simulink model "Quaternions_Method_main"  (R2021b)
settings: Solver=ode4  StartTime=0.0  StopTime=Time  FixedStep=1e-2  RelTol=1e-13  AbsTol=1e-8
values from neighbouring files (symbols this model uses):
  a = 8.6251e+06    (= 8625100)    [Main.m]
  c = 299792*10^3    (= 299792000)    [Main.m]
  e = 0.1195    [Main.m]
  f_mag = 18    [Main.m]
  H_0 = sqrt((g_1_0)^2 + (g_1_1)^2 + (h_1_1)^2)    [Main.m]
  i = 0.3815    [Main.m]
  MB = [2000; 0.3; 1; 0.12].*1e-2    [Main.m]
  muP = G*Mt    (= 398527110340000)    [Main.m]
  omega_0 = [om_x, om_y, om_z]    [Main.m]
  p_acc = 0.5    [Main.m]
  RD = 0.1*ones(1,10)    [Main.m]
  RS_MB = 0.5    [Main.m]
  RS_SP = 0.1    [Main.m]
  SP = [2000; 0.3; 1; 0.12].*1e-2    [Main.m]
  theta0 = 0    [Main.m]
  w_E = (2*pi)/(24*3600)    (= 7.27220521664e-05)    [Main.m]
undefined symbols (not defined in the file or in its folder): A_BN_0, A_rw, A_rw_star, k1, k2, magnitude, mr, sig_b, sig_n, T, t_sample
libraries: matrix_library x15, vrlib x8, simulink x2, simulink_extras x1
(part 5 of 5)

== system Quaternions_Method_main/Enviroment/Solar Radiation Perturbation/Sum forces/determine highlighted area/creazione della matrice che ha per colonne i vettori distanza tra il CM del MB e i centri geom delle aree illuminate dal sole /creazione raggi vettore tra CM MB e centro facce illuminate della faccia che ha come normale l'asse k/If Action Subsystem4 ==
  Areas_vect : Inport
  MB1 : Inport  Port=2
  Action Port : ActionPort  ActionPortLabel=if(u1<0 & u2>0)
  Add : Sum  Inputs=+|-
  Add1 : Sum  Inputs=+|-
  Add2 : Sum
  Demux : Demux  Outputs=3
  Demux1 : Demux  Outputs=3
  Demux2 : Demux
  Divide : Product  Inputs=*/
  Divide1 : Product  Inputs=*/
  Gain{,1..3} (4 alike) : Gain  Gain=1/2
  Gain4 : Gain  Gain=-1
  Ground : Ground
  Ground1 : Ground
  Mux : Mux  Inputs=3
  Mux1 : Mux  Inputs=3
  Reshape{,1..3} (4 alike) : Reshape  OutputDimensionality=Column vector (2-D)
  Terminator{,1..3,8..9} (6 alike) : Terminator
  r_cface_cluce_xneg_y_pos : Outport
  wires:
  Demux/2 -> Terminator8/1
  Demux/1 -> Terminator9/1
  Demux1/2 -> Terminator1/1
  Demux1/1 -> Terminator/1
  Add2/1 -> r_cface_cluce_xneg_y_pos/1
  Reshape3/1 -> Add2/2
  Reshape2/1 -> Add2/1
  Divide1/1 -> Gain3/1
  Reshape1/1 -> Demux1/1
  Gain2/1 -> Add1/1
  Gain3/1 -> Add1/2
  Demux1/3 -> Divide1/1
  Ground/1 -> Mux1/1, Mux1/3
  Mux1/1 -> Reshape3/1  "raggio vettore che collega il centro geom della faccia con il centro geom della faccia illuminata dal sole lungo j"
  Reshape/1 -> Demux/1
  Ground1/1 -> Mux/2, Mux/3
  Areas_vect/1 -> Reshape1/1, Reshape/1
  Gain/1 -> Add/1
  Demux/3 -> Divide/1
  Gain1/1 -> Add/2
  Mux/1 -> Reshape2/1  "raggio vettore che collega il centro geom della faccia con il centro geom della faccia illuminata dal sole lungo -i"
  Divide/1 -> Gain1/1
  [b_MB] -> Divide/2
  [a_MB] -> Gain/1
  Add/1 -> Gain4/1
  Gain4/1 -> Mux/1
  Add1/1 -> Mux1/2
  [b_MB] -> Gain2/1
  [a_MB] -> Divide1/2
  Demux2/1 -> Terminator2/1
  Demux2/2 -> [a_MB]
  MB1/1 -> Demux2/1
  Demux2/3 -> [b_MB]
  Demux2/4 -> Terminator3/1

== system Quaternions_Method_main/Enviroment/Solar Radiation Perturbation/Sum forces/determine highlighted area/creazione della matrice che ha per colonne i vettori distanza tra il CM del MB e i centri geom delle aree illuminate dal sole /creazione raggi vettore tra CM MB e centro facce illuminate della faccia che ha come normale l'asse k/If Action Subsystem5 ==
  Action Port : ActionPort  ActionPortLabel=else
  Constant : Constant  Value=[0;0;0]
  Out1 : Outport
  wires:
  Constant/1 -> Out1/1

== system Quaternions_Method_main/Enviroment/Solar Radiation Perturbation/Sum forces/determine highlighted area/creazione della matrice che ha per colonne i vettori distanza tra il CM del MB e i centri geom delle aree illuminate dal sole /creazione raggi vettore tra CM MB e centro facce illuminate della faccia che ha come normale l'asse k/If Action Subsystem6 ==
  Action Port : ActionPort  ActionPortLabel=else
  Constant : Constant  Value=[0;0;0]
  Out1 : Outport
  wires:
  Constant/1 -> Out1/1

== system Quaternions_Method_main/Enviroment/Solar Radiation Perturbation/Sum forces/determine highlighted area/creazione della matrice che ha per colonne i vettori distanza tra il CM del MB e i centri geom delle aree illuminate dal sole /creazione raggi vettore tra CM MB e centro facce illuminate della faccia che ha come normale l'asse k/If Action Subsystem7 ==
  Action Port : ActionPort  ActionPortLabel=else
  Constant : Constant  Value=[0;0;0]
  Out1 : Outport
  wires:
  Constant/1 -> Out1/1

== system Quaternions_Method_main/Enviroment/Solar Radiation Perturbation/Sum forces/determine highlighted area/creazione della matrice che ha per colonne i vettori distanza tra il CM del MB e i centri geom delle aree illuminate dal sole /creazione raggi vettore tra CM MB e centro facce illuminate della faccia che ha come normale l'asse k/creating distance between cm MB and centro geom lato1 ==
  MB : Inport
  Demux : Demux
  Ground : Ground
  Mux : Mux  Inputs=3
  Reshape : Reshape  OutputDimensionality=Column vector (2-D)
  Terminator : Terminator
  Terminator2 : Terminator
  Terminator3 : Terminator
  Out1 : Outport
  wires:
  Reshape/1 -> Out1/1
  Mux/1 -> Reshape/1
  MB/1 -> Demux/1
  Demux/1 -> Terminator/1
  Demux/2 -> Mux/1
  Demux/3 -> Terminator2/1
  Ground/1 -> Mux/2, Mux/3
  Demux/4 -> Terminator3/1

== matlab function Quaternions_Method_main/Attitude determination/MATLAB Function ==
  data: K input; V output; D output
function [V, D] = fcn(K)
[V,D] = eig(K);
end

== matlab function Quaternions_Method_main/Enviroment/Magnetic torque /Magnetic torque in body frame/MATLAB Function ==
  data: teta0 input; R input; r_LVLH input; th input; B_N output
function B_N = fcn(teta0, R, r_LVLH, th)
%% First thing is to define the vector containing all the polynimials up to the 4th order
fun1 = 1;
fun2 = @(th) th;
fun3 = @(th) ((3*th^2)-1)/2;
fun4 = @(th) ((5*th^3)-(3*th))/2;

P1 = 1;
P2 = fsolve(fun2, teta0);
P3 = fsolve(fun3, teta0);
P4 = fsolve(fun4, teta0);

% Computing the derivatives of the P polynomials
fun1_der = 0;
fun2_der = 1;
fun3_der = @(th) 3*th;
fun4_der = @(th) ((15*th^2)-3)/2;

P1_der = 0;
P2_der = 1;
P3_der = fsolve(fun3_der, teta0);
P4_der = fsolve(fun4_der, teta0);

r = norm(r_LVLH);
% Defining the order of the approximation k 
k = 4;

% Defining the matrices containing the coefficients needed to make the
% approximation model IGRF2000 (following the tables on the slide number 5 of the
% pack of slides number 8)
g = 1e9*[-29615 -1728 0 0 0; ...
                      -2267 3072 1672 0 0; ...
                     1341 -2290 1253 715 0; ...
                     935 787 251 -405 110]; %[T]
h = 1e9*[0 5186 0 0 0; ...
                     0 -2478 -458 0 0; ...
                     0 -227 296 -492 0; ...
                     0 272 -232 119 -304]; %[T]

% Computing the right ascension alpha, the declination delta, the longitude lon and the co-latitude phi
delta = asin(r_LVLH(3)/r); %[rad]
if(r_LVLH(2)/r > 0)
    alpha = acos((r_LVLH(1)/r)/cos(delta)); %[rad]
else 
    alpha = 2*pi -  acos((r_LVLH(1)/r)/cos(delta)); %[rad]
end
lat = -delta; %[rad]
phi = pi - lat; %[rad]
om_E = deg2rad(15.04)/3600; 
Gren_lon = om_E*t;
lon = (alpha - Gren_lon);

% Computing the for cicle to obtain components of B in r, th, phi RF
b_r = [];
b_th = [];
b_phi = [];

for n = 1:k
    for m = 1:(n+1)
        P_mat = (2*factorial(n-m))/factorial(n+m)*[P1, P1, P1, P1; P2, P2, P2, P2; P3, P3, P3, P3; P4, P4, P4, P4];
        P_matder = (2*factorial(n-m))/factorial(n+m)*[P1_der, P1_der, P1_der, P1_der; P2_der, P2_der, P2_der, P2_der; P3_der, P3_der, P3_der, P3_der; P4_der, P4_der, P4_der, P4_der];
        b_r = (R/r)^n+2*(n+1)*((g(n, m)*cos(m*phi)+h(n,m)*sin(m*phi))*P_mat(n,m));
        b_th = -(R/r)^(n+2)*((g(n, m)*cos(m*phi)+h(n,m)*sin(m*phi))*P_matder(n,m));
        b_phi = -1/sin(th)*((R/r)^(n+2))*((-g(n,m)*sin(m*phi) + h(n,m)*cos(m*phi))*P_mat(n,m));

        % Computing the magnetic torque in the inertial frame 
        b1 = (b_r*cos(delta)+b_th*sin(delta))*cos(alpha)-b_phi*sin(alpha);
        b2 = (b_r*cos(delta)+b_th*sin(delta))*sin(alpha)+b_phi*cos(alpha);
        b3 = b_r*sin(delta)-b_th*cos(delta);
    end
end
B_N = [b1; b2; b3];


end
